simulink model "adrc_speed_controller_wrapper"  (R2026a)
settings: Solver=FixedStepDiscrete  FixedStep=0.0005
settings Model: Creator=ASUS  LastModifiedBy=ASUS
settings HardwareCC: ProdLargestAtomicInteger=Long  ProdLargestAtomicFloat=Double  ProdHWDeviceType=ARM Compatible->ARM Cortex
settings RTWCC: SystemTargetFile=ert.tlc  GenCodeOnly=on  Description=Embedded Coder
settings ERTTargetCC: GenerateSampleERTMain=on  SupportComplex=off

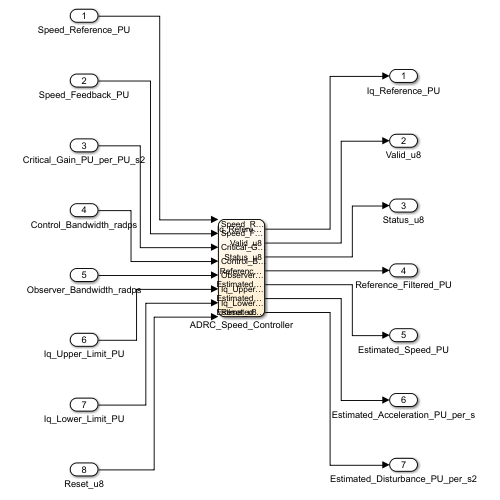
[thumbnail: Simulink's stored preview of the top-level diagram]
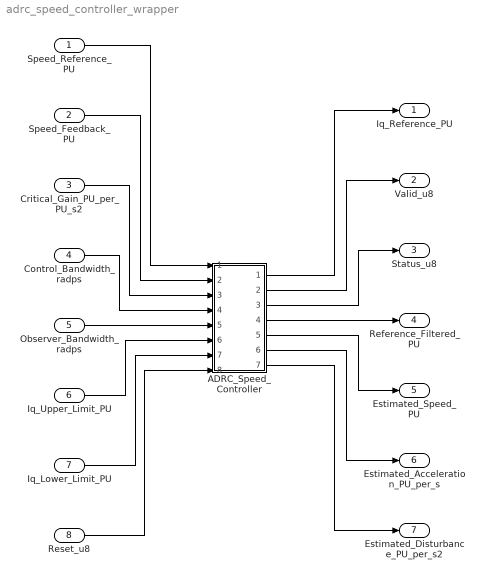
== system adrc_speed_controller_wrapper ==
  Speed_Reference_PU : Inport  OutDataTypeStr=single  SampleTime=0.0005
  Speed_Feedback_PU : Inport  Port=2  OutDataTypeStr=single  SampleTime=0.0005
  Critical_Gain_PU_per_PU_s2 : Inport  Port=3  OutDataTypeStr=single  SampleTime=0.0005
  Control_Bandwidth_radps : Inport  Port=4  OutDataTypeStr=single  SampleTime=0.0005
  Observer_Bandwidth_radps : Inport  Port=5  OutDataTypeStr=single  SampleTime=0.0005
  Iq_Upper_Limit_PU : Inport  Port=6  OutDataTypeStr=single  SampleTime=0.0005
  Iq_Lower_Limit_PU : Inport  Port=7  OutDataTypeStr=single  SampleTime=0.0005
  Reset_u8 : Inport  Port=8  OutDataTypeStr=uint8  SampleTime=0.0005
  ADRC_Speed_Controller : Stateflow chart  TreatAsAtomicUnit=on
  Iq_Reference_PU : Outport  OutDataTypeStr=single
  Valid_u8 : Outport  Port=2  OutDataTypeStr=uint8
  Status_u8 : Outport  Port=3  OutDataTypeStr=uint8
  Reference_Filtered_PU : Outport  Port=4  OutDataTypeStr=single
  Estimated_Speed_PU : Outport  Port=5  OutDataTypeStr=single
  Estimated_Acceleration_PU_per_s : Outport  Port=6  OutDataTypeStr=single
  Estimated_Disturbance_PU_per_s2 : Outport  Port=7  OutDataTypeStr=single
  wires:
  ADRC_Speed_Controller/7(Estimated_Disturbance_PU_per_s2) -> Estimated_Disturbance_PU_per_s2/1
  ADRC_Speed_Controller/6(Estimated_Acceleration_PU_per_s) -> Estimated_Acceleration_PU_per_s/1
  ADRC_Speed_Controller/5(Estimated_Speed_PU) -> Estimated_Speed_PU/1
  ADRC_Speed_Controller/4(Reference_Filtered_PU) -> Reference_Filtered_PU/1
  ADRC_Speed_Controller/3(Status_u8) -> Status_u8/1
  ADRC_Speed_Controller/2(Valid_u8) -> Valid_u8/1
  ADRC_Speed_Controller/1(Iq_Reference_PU) -> Iq_Reference_PU/1
  Reset_u8/1 -> ADRC_Speed_Controller/8(Reset_u8)
  Iq_Lower_Limit_PU/1 -> ADRC_Speed_Controller/7(Iq_Lower_Limit_PU)
  Iq_Upper_Limit_PU/1 -> ADRC_Speed_Controller/6(Iq_Upper_Limit_PU)
  Observer_Bandwidth_radps/1 -> ADRC_Speed_Controller/5(Observer_Bandwidth_radps)
  Control_Bandwidth_radps/1 -> ADRC_Speed_Controller/4(Control_Bandwidth_radps)
  Critical_Gain_PU_per_PU_s2/1 -> ADRC_Speed_Controller/3(Critical_Gain_PU_per_PU_s2)
  Speed_Feedback_PU/1 -> ADRC_Speed_Controller/2(Speed_Feedback_PU)
  Speed_Reference_PU/1 -> ADRC_Speed_Controller/1(Speed_Reference_PU)

== stateflow chart adrc_speed_controller_wrapper/ADRC_Speed_Controller ==
  state Run
    en:
    referenceFilterState = single(0);
    observerState0 = single(0);
    observerState1 = single(0);
    observerState2 = single(0);
    [Iq_Reference_PU, Valid_u8, Status_u8, Reference_Filtered_PU, referenceFilterState, observerState0, observerState1, observerState2] = adrcStep(Speed_Reference_PU, Speed_Feedback_PU, Critical_Gain_PU_per_PU_s2, Control_Bandwidth_radps, Observer_Bandwidth_radps, Iq_Upper_Limit_PU, Iq_Lower_Limit_PU, Reset_u8, referenceFilterState, observerState0, observerState1, observerState2);
    Estimated_Speed_PU = observerState0;
    Estimated_Acceleration_PU_per_s = observerState1;
    Estimated_Disturbance_PU_per_s2 = observerState2;
    du:
    [Iq_Reference_PU, Valid_u8, Status_u8, Reference_Filtered_PU, referenceFilterState, observerState0, observerState1, observerState2] = adrcStep(Speed_Reference_PU, Speed_Feedback_PU, Critical_Gain_PU_per_PU_s2, Control_Bandwidth_radps, Observer_Bandwidth_radps, Iq_Upper_Limit_PU, Iq_Lower_Limit_PU, Reset_u8, referenceFilterState, observerState0, observerState1, observerState2);
    Estimated_Speed_PU = observerState0;
    Estimated_Acceleration_PU_per_s = observerState1;
    Estimated_Disturbance_PU_per_s2 = observerState2;
  (default) -> Run
  data: referencePU function_input; measuredPU function_input; criticalGain function_input; controlBandwidth function_input; observerBandwidth function_input; upperLimit function_input; lowerLimit function_input; reset function_input; referenceFilterStateIn function_input; state0 function_input; state1 function_input; state2 function_input; iqReferencePU function_output; valid function_output; status function_output; referenceFilteredPU function_output; nextReferenceFilterState function_output; nextState0 function_output; nextState1 function_output; nextState2 function_output; Speed_Reference_PU input single; Speed_Feedback_PU input single; Critical_Gain_PU_per_PU_s2 input single; Control_Bandwidth_radps input single; Observer_Bandwidth_radps input single; Iq_Upper_Limit_PU input single; Iq_Lower_Limit_PU input single; Reset_u8 input uint8; Iq_Reference_PU output single; Valid_u8 output uint8; Status_u8 output uint8; Reference_Filtered_PU output single; Estimated_Speed_PU output single; Estimated_Acceleration_PU_per_s output single; Estimated_Disturbance_PU_per_s2 output single; referenceFilterState local single; observerState0 local single; observerState1 local single; observerState2 local single
  function [iqReferencePU, valid, status, referenceFilteredPU, nextReferenceFilterState, nextState0, nextState1, nextState2] = adrcStep(referencePU, measuredPU, criticalGain, controlBandwidth, observerBandwidth, upperLimit, lowerLimit, reset, referenceFilterStateIn, state0, state1, state2):
    | function [iqReferencePU, valid, status, referenceFilteredPU, nextReferenceFilterState, nextState0, nextState1, nextState2] = adrcStep(referencePU, measuredPU, criticalGain, controlBandwidth, observerBandwidth, upperLimit, lowerLimit, reset, referenceFilterStateIn, state0, state1, state2)
    | %#codegen
    | Ts = single(0.0005);
    | filterGain = single(0.1);
    | iqReferencePU = single(0);
    | valid = uint8(0);
    | status = uint8(0);
    | referenceFilteredPU = single(0);
    | nextReferenceFilterState = single(0);
    | nextState0 = single(0);
    | nextState1 = single(0);
    | nextState2 = single(0);
    | 
    | if reset ~= uint8(0)
    |     return;
    | end
    | 
    | if ~(isfinite(referencePU) && isfinite(measuredPU) && isfinite(criticalGain) && isfinite(controlBandwidth) && isfinite(observerBandwidth) && isfinite(upperLimit) && isfinite(lowerLimit))
    |     status = uint8(3);
    |     return;
    | end
    | 
    | if (criticalGain <= single(0)) || (controlBandwidth <= single(0)) || (observerBandwidth <= single(0)) || (lowerLimit > upperLimit)
    |     status = uint8(2);
    |     return;
    | end
    | 
    | observerPole = exp(-observerBandwidth * Ts);
    | oneMinusPole = single(1) - observerPole;
    | observerGain0 = single(1) - observerPole * observerPole * observerPole;
    | observerGain1 = (single(1.5) / Ts) * oneMinusPole * oneMinusPole * (single(1) + observerPole);
    | observerGain2 = oneMinusPole * oneMinusPole * oneMinusPole / (Ts * Ts);
    | controlGain = controlBandwidth * controlBandwidth;
    | dampingGain = single(2) * controlBandwidth;
    | inputGain0 = single(0.5) * Ts * Ts * criticalGain;
    | inputGain1 = Ts * criticalGain;
    | inverseCriticalGain = single(1) / criticalGain;
    | 
    | if ~(isfinite(observerPole) && isfinite(observerGain0) && isfinite(observerGain1) && isfinite(observerGain2) && isfinite(controlGain) && isfinite(dampingGain) && isfinite(inputGain0) && isfinite(inputGain1) && isfinite(inverseCriticalGain))
    |     status = uint8(3);
    |     return;
    | end
    | 
    | referenceFilteredPU = referenceFilterStateIn + filterGain * (referencePU - referenceFilterStateIn);
    | nextReferenceFilterState = referenceFilteredPU;
    | observerError = measuredPU - state0;
    | correctedState0 = state0 + observerGain0 * observerError;
    | correctedState1 = state1 + observerGain1 * observerError;
    | correctedState2 = state2 + observerGain2 * observerError;
    | iqReferencePU = ((referenceFilteredPU - correctedState0) * controlGain - dampingGain * correctedState1 - correctedState2) * inverseCriticalGain;
    | 
    | if iqReferencePU > upperLimit
    |     iqReferencePU = upperLimit;
    | elseif iqReferencePU < lowerLimit
    |     iqReferencePU = lowerLimit;
    | end
    | 
    | nextState0 = correctedState0 + Ts * correctedState1 + single(0.5) * Ts * Ts * correctedState2 + inputGain0 * iqReferencePU;
    | nextState1 = correctedState1 + Ts * correctedState2 + inputGain1 * iqReferencePU;
    | nextState2 = correctedState2;
    | 
    | if ~(isfinite(referenceFilteredPU) && isfinite(iqReferencePU) && isfinite(nextState0) && isfinite(nextState1) && isfinite(nextState2))
    |     iqReferencePU = single(0);
    |     referenceFilteredPU = single(0);
    |     nextReferenceFilterState = single(0);
    |     nextState0 = single(0);
    |     nextState1 = single(0);
    |     nextState2 = single(0);
    |     status = uint8(3);
    |     return;
    | end
    | 
    | valid = uint8(1);
    | status = uint8(1);
    | end
